simulink model "segway_linmod_no_L"  (R2023a)
settings: Solver=VariableStepAuto  StartTime=0.0  StopTime=10.0  RelTol=1e-3
undefined symbols (not defined in the file or in its folder): Cinp, Cout, Cr2w, Cw2r, p
libraries: cstblocks x1
settings Model: Creator=Michael Peter  LastModifiedBy=Michael Peter

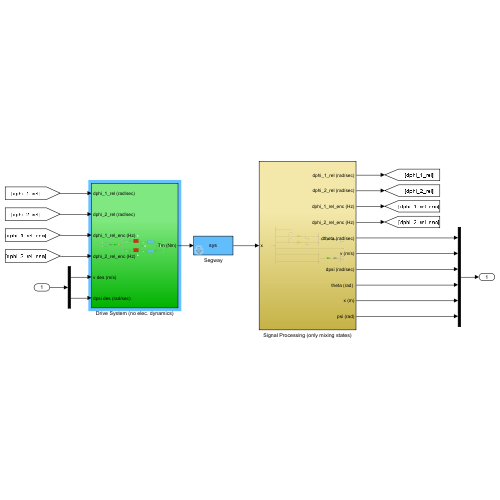
[thumbnail: Simulink's stored preview of the top-level diagram]
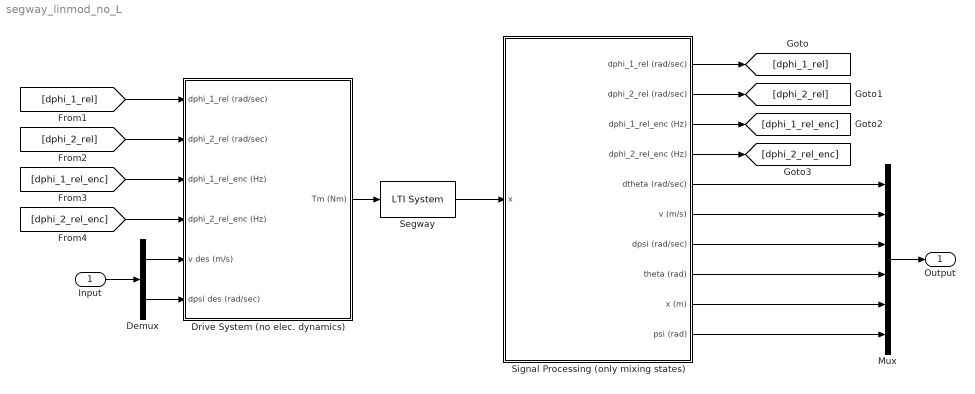
== system segway_linmod_no_L ==
  Input : Inport
  Demux : Demux  Outputs=2
  Drive System (no elec. dynamics) : Subsystem
  Mux : Mux  Inputs=6
  Segway : cstblocks/LTI System  sys=sys  IC=x0
  Signal Processing (only mixing states) : Subsystem
  Output : Outport
  wires:
  Signal Processing (only mixing states)/1(dphi_1_rel (rad/sec)) -> [dphi_1_rel]
  Signal Processing (only mixing states)/3(dphi_1_rel_enc (Hz)) -> [dphi_1_rel_enc]
  Signal Processing (only mixing states)/2(dphi_2_rel (rad/sec)) -> [dphi_2_rel]
  Segway/1 -> Signal Processing (only mixing states)/1(x)
  Signal Processing (only mixing states)/4(dphi_2_rel_enc (Hz)) -> [dphi_2_rel_enc]
  Signal Processing (only mixing states)/8("theta (rad) ") -> Mux/4
  Signal Processing (only mixing states)/5(dtheta (rad/sec)) -> Mux/1
  Signal Processing (only mixing states)/7(dpsi (rad/sec)) -> Mux/3
  Signal Processing (only mixing states)/10(psi (rad)) -> Mux/6
  Mux/1 -> Output/1
  Signal Processing (only mixing states)/9(x (m)) -> Mux/5
  Signal Processing (only mixing states)/6(v (m/s)) -> Mux/2
  [dphi_2_rel_enc] -> Drive System (no elec. dynamics)/4(dphi_2_rel_enc (Hz))
  [dphi_1_rel_enc] -> Drive System (no elec. dynamics)/3(dphi_1_rel_enc (Hz))
  Input/1 -> Demux/1
  Demux/1 -> Drive System (no elec. dynamics)/5(v des (m/s))
  [dphi_2_rel] -> Drive System (no elec. dynamics)/2(dphi_2_rel (rad/sec))
  [dphi_1_rel] -> Drive System (no elec. dynamics)/1(dphi_1_rel (rad/sec))
  Drive System (no elec. dynamics)/1(Tm (Nm)) -> Segway/1
  Demux/2 -> Drive System (no elec. dynamics)/6(dpsi des (rad/sec))

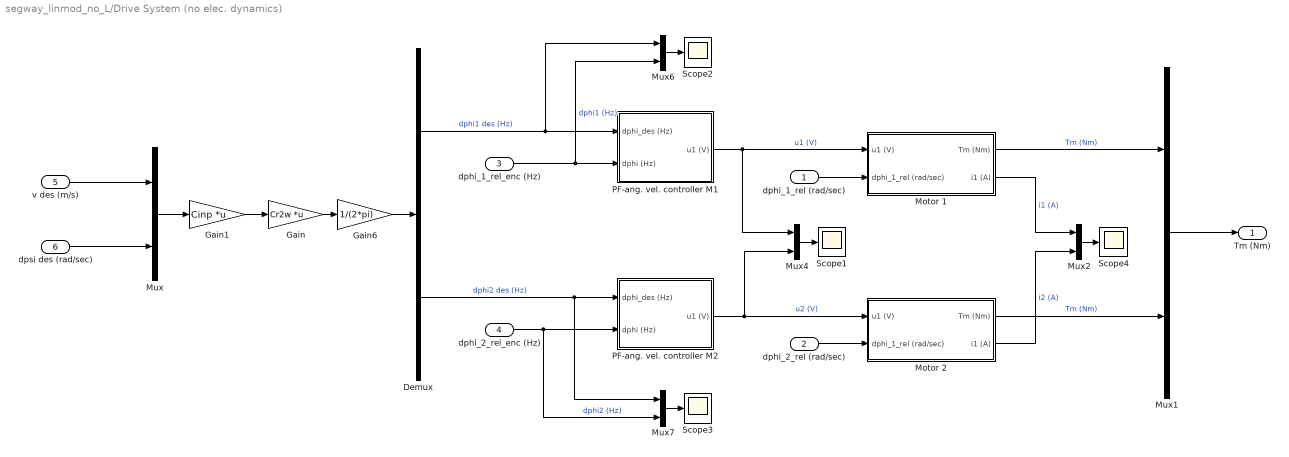
== system segway_linmod_no_L/Drive System (no elec. dynamics) ==
  dphi_1_rel (rad/sec) : Inport
  dphi_2_rel (rad/sec) : Inport  Port=2
  dphi_1_rel_enc (Hz) : Inport  Port=3
  dphi_2_rel_enc (Hz) : Inport  Port=4
  v des (m/s) : Inport  Port=5
  dpsi des (rad/sec) : Inport  Port=6
  Demux : Demux  Outputs=2
  Gain : Gain  Gain=Cr2w  Multiplication=Matrix(K*u)
  Gain1 : Gain  Gain=Cinp  Multiplication=Matrix(K*u)
  Gain6 : Gain  Gain=1/(2*pi)
  Motor 1 : Subsystem
  Motor 2 : Subsystem
  Mux{,1..2,4,6..7} (6 alike) : Mux  Inputs=2
  PF-ang. vel. controller M1 : Subsystem
  PF-ang. vel. controller M2 : Subsystem
  Scope{1..4} (4 alike) : Scope
  Tm (Nm) : Outport
  wires:
  dphi_1_rel_enc (Hz)/1 -> PF-ang. vel. controller M1/2(dphi (Hz)), Mux6/2  "dphi1 (Hz)"
  dphi_1_rel (rad/sec)/1 -> Motor 1/2(dphi_1_rel (rad/sec))
  Motor 2/2(i1 (A)) -> Mux2/2  "i2 (A)"
  Mux4/1 -> Scope1/1
  Demux/1 -> PF-ang. vel. controller M1/1(dphi_des (Hz)), Mux6/1  "dphi1 des (Hz)"
  Demux/2 -> PF-ang. vel. controller M2/1(dphi_des (Hz)), Mux7/1  "dphi2 des (Hz)"
  Mux7/1 -> Scope3/1
  PF-ang. vel. controller M1/1(u1 (V)) -> Mux4/1, Motor 1/1(u1 (V))  "u1 (V)"
  Motor 1/1(Tm (Nm)) -> Mux1/1  "Tm (Nm)"
  dphi_2_rel_enc (Hz)/1 -> PF-ang. vel. controller M2/2(dphi (Hz)), Mux7/2  "dphi2 (Hz)"
  PF-ang. vel. controller M2/1(u1 (V)) -> Motor 2/1(u1 (V)), Mux4/2  "u2 (V)"
  Mux6/1 -> Scope2/1
  Motor 2/1(Tm (Nm)) -> Mux1/2  "Tm (Nm)"
  Mux1/1 -> Tm (Nm)/1
  dphi_2_rel (rad/sec)/1 -> Motor 2/2(dphi_1_rel (rad/sec))
  Motor 1/2(i1 (A)) -> Mux2/1  "i1 (A)"
  Mux2/1 -> Scope4/1
  dpsi des (rad/sec)/1 -> Mux/2
  v des (m/s)/1 -> Mux/1
  Mux/1 -> Gain1/1
  Gain6/1 -> Demux/1
  Gain/1 -> Gain6/1
  Gain1/1 -> Gain/1

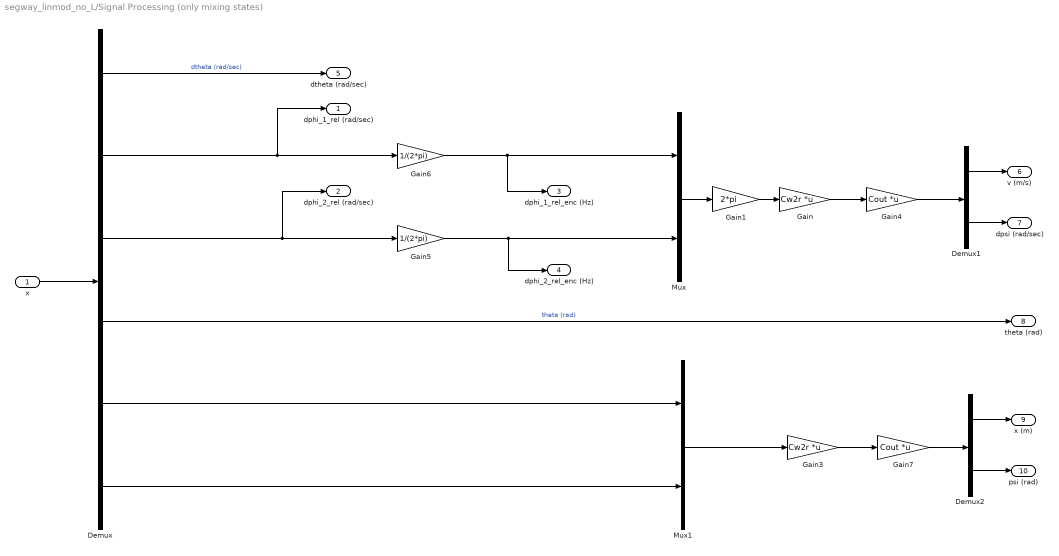
== system segway_linmod_no_L/Signal Processing (only mixing states) ==
  x : Inport
  Demux : Demux  Outputs=6
  Demux1 : Demux  Outputs=2
  Demux2 : Demux  Outputs=2
  Gain : Gain  Gain=Cw2r  Multiplication=Matrix(K*u)
  Gain1 : Gain  Gain=2*pi
  Gain3 : Gain  Gain=Cw2r  Multiplication=Matrix(K*u)
  Gain4 : Gain  Gain=Cout  Multiplication=Matrix(K*u)
  Gain5 : Gain  Gain=1/(2*pi)
  Gain6 : Gain  Gain=1/(2*pi)
  Gain7 : Gain  Gain=Cout  Multiplication=Matrix(K*u)
  Mux : Mux  Inputs=2
  Mux1 : Mux  Inputs=2
  dphi_1_rel (rad/sec) : Outport
  dphi_2_rel (rad/sec) : Outport  Port=2
  dphi_1_rel_enc (Hz) : Outport  Port=3
  dphi_2_rel_enc (Hz) : Outport  Port=4
  dtheta (rad/sec) : Outport  Port=5
  v (m/s) : Outport  Port=6
  dpsi (rad/sec) : Outport  Port=7
  "theta (rad) " : Outport  Port=8
  x (m) : Outport  Port=9
  psi (rad) : Outport  Port=10
  wires:
  Demux/1 -> dtheta (rad/sec)/1  "dtheta (rad/sec)"
  Demux/2 -> Gain6/1, dphi_1_rel (rad/sec)/1
  Demux/3 -> Gain5/1, dphi_2_rel (rad/sec)/1
  Demux/4 -> "theta (rad) "/1  "theta (rad)"
  x/1 -> Demux/1
  Mux/1 -> Gain1/1
  Gain6/1 -> Mux/1, dphi_1_rel_enc (Hz)/1
  Gain5/1 -> Mux/2, dphi_2_rel_enc (Hz)/1
  Gain1/1 -> Gain/1
  Demux1/1 -> v (m/s)/1
  Demux1/2 -> dpsi (rad/sec)/1
  Mux1/1 -> Gain3/1
  Demux2/2 -> psi (rad)/1
  Demux2/1 -> x (m)/1
  Gain7/1 -> Demux2/1
  Gain3/1 -> Gain7/1
  Gain/1 -> Gain4/1
  Gain4/1 -> Demux1/1
  Demux/6 -> Mux1/2
  Demux/5 -> Mux1/1

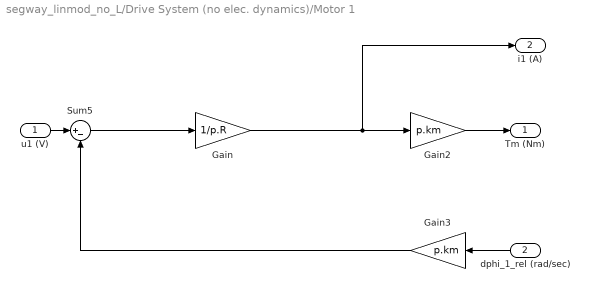
== system segway_linmod_no_L/Drive System (no elec. dynamics)/Motor 1 ==
  u1 (V) : Inport
  dphi_1_rel (rad/sec) : Inport  Port=2
  Gain : Gain  Gain=1/p.R
  Gain2 : Gain  Gain=p.km
  Gain3 : Gain  Gain=p.km
  Sum5 : Sum  Inputs=|+-
  Tm (Nm) : Outport
  i1 (A) : Outport  Port=2
  wires:
  Gain/1 -> i1 (A)/1, Gain2/1
  Gain3/1 -> Sum5/2
  u1 (V)/1 -> Sum5/1
  Sum5/1 -> Gain/1
  dphi_1_rel (rad/sec)/1 -> Gain3/1
  Gain2/1 -> Tm (Nm)/1

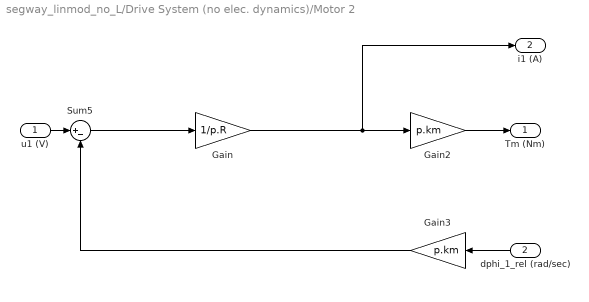
== system segway_linmod_no_L/Drive System (no elec. dynamics)/Motor 2 ==
  u1 (V) : Inport
  dphi_1_rel (rad/sec) : Inport  Port=2
  Gain : Gain  Gain=1/p.R
  Gain2 : Gain  Gain=p.km
  Gain3 : Gain  Gain=p.km
  Sum5 : Sum  Inputs=|+-
  Tm (Nm) : Outport
  i1 (A) : Outport  Port=2
  wires:
  Gain2/1 -> Tm (Nm)/1
  dphi_1_rel (rad/sec)/1 -> Gain3/1
  Sum5/1 -> Gain/1
  u1 (V)/1 -> Sum5/1
  Gain3/1 -> Sum5/2
  Gain/1 -> Gain2/1, i1 (A)/1

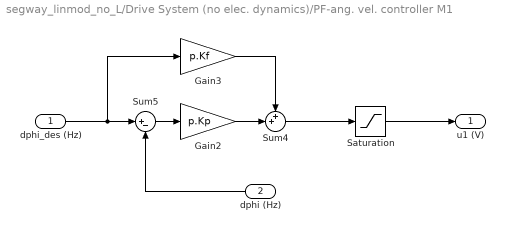
== system segway_linmod_no_L/Drive System (no elec. dynamics)/PF-ang. vel. controller M1 ==
  dphi_des (Hz) : Inport
  dphi (Hz) : Inport  Port=2
  Gain2 : Gain  Gain=p.Kp
  Gain3 : Gain  Gain=p.Kf
  Saturation : Saturate  UpperLimit=p.u_max  LowerLimit=p.u_min
  Sum4 : Sum  Inputs=++|
  Sum5 : Sum  Inputs=|+-
  u1 (V) : Outport
  wires:
  Sum5/1 -> Gain2/1
  dphi_des (Hz)/1 -> Gain3/1, Sum5/1
  dphi (Hz)/1 -> Sum5/2
  Gain3/1 -> Sum4/1
  Gain2/1 -> Sum4/2
  Sum4/1 -> Saturation/1
  Saturation/1 -> u1 (V)/1

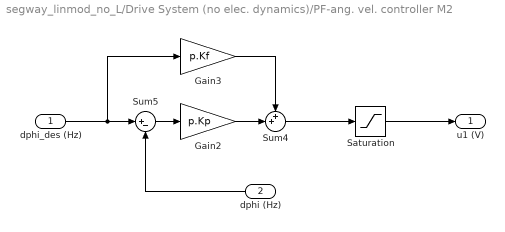
== system segway_linmod_no_L/Drive System (no elec. dynamics)/PF-ang. vel. controller M2 ==
  dphi_des (Hz) : Inport
  dphi (Hz) : Inport  Port=2
  Gain2 : Gain  Gain=p.Kp
  Gain3 : Gain  Gain=p.Kf
  Saturation : Saturate  UpperLimit=p.u_max  LowerLimit=p.u_min
  Sum4 : Sum  Inputs=++|
  Sum5 : Sum  Inputs=|+-
  u1 (V) : Outport
  wires:
  Sum5/1 -> Gain2/1
  dphi_des (Hz)/1 -> Gain3/1, Sum5/1
  dphi (Hz)/1 -> Sum5/2
  Gain3/1 -> Sum4/1
  Gain2/1 -> Sum4/2
  Sum4/1 -> Saturation/1
  Saturation/1 -> u1 (V)/1
